simulink subsystem "subsistema_motores"  (R2023b)
settings: Solver=VariableStepAuto  StartTime=0.0  StopTime=10.0  RelTol=1e-3
libraries: arduinolib x6
settings Model: Creator=Usuario_UMA  LastModifiedBy=Usuario_UMA

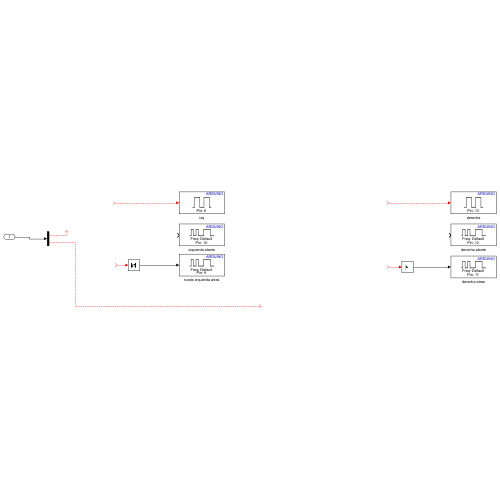
[thumbnail: Simulink's stored preview of the top-level diagram]
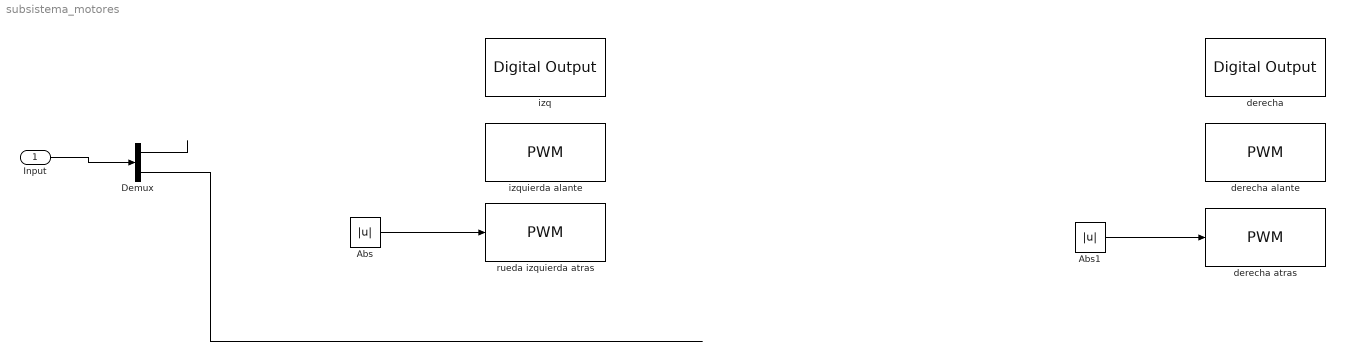
== system subsistema_motores ==
  Input : Inport
  Abs : Abs  SaturateOnIntegerOverflow=off
  Abs1 : Abs  SaturateOnIntegerOverflow=off
  Demux : Demux  Outputs=2
  derecha : arduinolib/Digital Output  pinNumber=13  Direction=output  blockPlatform=arduino
  derecha alante : arduinolib/PWM  pinNumber=12  frequencyType=Default  desiredFrequency=490.2  achievableFrequency=490.2
  derecha atras : arduinolib/PWM  pinNumber=11  frequencyType=Default  desiredFrequency=490.2  achievableFrequency=490.2
  izq : arduinolib/Digital Output  pinNumber=8  Direction=output  blockPlatform=arduino
  izquierda alante : arduinolib/PWM  pinNumber=10  frequencyType=Default  desiredFrequency=490.2  achievableFrequency=490.2
  rueda izquierda atras : arduinolib/PWM  pinNumber=9  frequencyType=Default  desiredFrequency=490.2  achievableFrequency=490.2
  wires:
  Demux/2 -> ?
  ? -> Abs1/1
  ? -> izq/1
  Demux/1 -> ?
  Abs1/1 -> derecha atras/1
  ? -> derecha/1
  ? -> Abs/1
  Abs/1 -> rueda izquierda atras/1
  Input/1 -> Demux/1
